simulink model "plant_test"  (R2023b)
settings: Solver=VariableStepAuto  StartTime=0.0  StopTime=t_end  RelTol=1e-3
values from neighbouring files (symbols this model uses):
  param = plant_param()    [plot_bode.m]    (also in plot_impulse.m; plot_initial.m)
  Ts = (2*pi)/(100*w)    [plot_bode.m]    (also in plot_impulse.m = 0.001; plot_initial.m = 0.001)
  w = w_vec(i)    [plot_bode.m]
  x0 = [0;0;10e3;10e3]    [plot_initial.m]
undefined symbols (not defined in the file or in its folder): ue, xe
libraries: fl_lib x32, nesl_utility x14, simulink x4
(part 1 of 3)
settings Model: Creator=MPC5  LastModifiedBy=MPC5

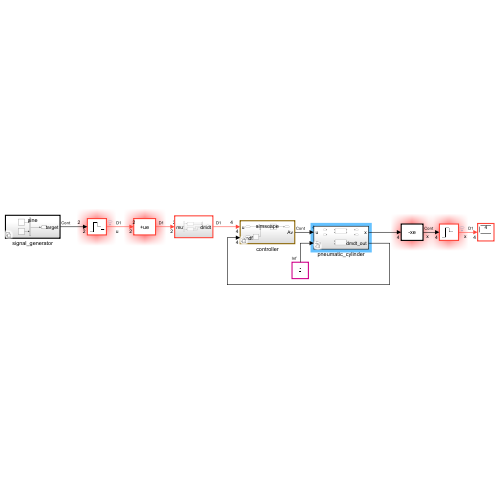
[thumbnail: Simulink's stored preview of the top-level diagram]
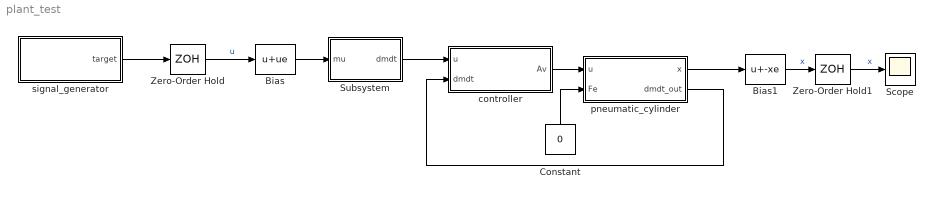
== system plant_test ==
  Bias : Bias  Bias=ue  SaturateOnIntegerOverflow=off
  Bias1 : Bias  Bias=-xe  SaturateOnIntegerOverflow=off
  Constant : Constant  Value=0
  Scope : Scope
  Subsystem : Subsystem
  Zero-Order Hold : ZeroOrderHold  SampleTime=Ts
  Zero-Order Hold1 : ZeroOrderHold  SampleTime=Ts
  controller : Subsystem  Variant=on
  pneumatic_cylinder : Subsystem  Variant=on
  signal_generator : Subsystem  Variant=on
  wires:
  Zero-Order Hold/1 -> Bias/1  "u"
  Bias/1 -> Subsystem/1(mu)
  Subsystem/1(dmdt) -> controller/1(u)
  pneumatic_cylinder/2(dmdt_out) -> controller/2(dmdt)
  controller/1(Av) -> pneumatic_cylinder/1(u)
  Constant/1 -> pneumatic_cylinder/2(Fe)
  pneumatic_cylinder/1(x) -> Bias1/1
  Zero-Order Hold1/1 -> Scope/1  "x"
  signal_generator/1(target) -> Zero-Order Hold/1
  Bias1/1 -> Zero-Order Hold1/1  "x"

== system plant_test/Subsystem ==
  mu : Inport
  Demux : Demux  Outputs=2
  Mux : Mux
  muc_to_dmcdt : Subsystem
  muh_to_dmhdt : Subsystem
  dmdt : Outport
  wires:
  Demux/1 -> muc_to_dmcdt/1(mu)
  muc_to_dmcdt/1(dmdt_in) -> Mux/1
  muc_to_dmcdt/2(dmdt_out) -> Mux/2
  Demux/2 -> muh_to_dmhdt/1(mu)
  muh_to_dmhdt/1(dmdt_in) -> Mux/3
  muh_to_dmhdt/2(dmdt_out) -> Mux/4
  mu/1 -> Demux/1
  Mux/1 -> dmdt/1

== system plant_test/controller ==
  u : Inport
  dmdt : Inport  Port=2
  ode : Subsystem  VariantControl="plant_model_type==\"ode\""
  simscape : Subsystem  VariantControl="plant_model_type==\"simscape\""
  Av : Outport

== system plant_test/pneumatic_cylinder ==
  u : Inport
  Fe : Inport  Port=2
  ode : Subsystem  VariantControl="plant_model_type==\"ode\""
  simscape : Subsystem  VariantControl="plant_model_type==\"simscape\""
  x : Outport
  dmdt_out : Outport  Port=2

== system plant_test/signal_generator ==
  impulse : Subsystem  VariantControl="input_signal_type==\"impulse\""
  sine : Subsystem  VariantControl="input_signal_type==\"sine\""
  zero : Subsystem  VariantControl="input_signal_type==\"zero\""
  target : Outport

== system plant_test/Subsystem/muc_to_dmcdt ==
  note: Pa <= P <= Ps
  mu : Inport
  Constant : Constant  Value=0
  Gain : Gain  Gain=-1
  Gain3 : Gain  Gain=1/param.alpha_in
  Gain4 : Gain  Gain=1/param.alpha_out
  Max : MinMax  Function=max  Inputs=2
  Min : MinMax  Function=max  Inputs=2
  dmdt_in : Outport
  dmdt_out : Outport  Port=2
  wires:
  Gain3/1 -> Max/1
  Constant/1 -> Max/2, Min/1
  Gain/1 -> Gain4/1
  mu/1 -> Gain3/1, Gain/1  "mu"
  Gain4/1 -> Min/2
  Min/1 -> dmdt_out/1  "dmdt_out"
  Max/1 -> dmdt_in/1  "dmdt_in"

== system plant_test/Subsystem/muh_to_dmhdt ==
  note: Pa <= P <= Ps
  mu : Inport
  Constant : Constant  Value=0
  Gain : Gain  Gain=-1
  Gain3 : Gain  Gain=1/param.alpha_in
  Gain4 : Gain  Gain=1/param.alpha_out
  Max : MinMax  Function=max  Inputs=2
  Min : MinMax  Function=max  Inputs=2
  dmdt_in : Outport
  dmdt_out : Outport  Port=2
  wires:
  Gain3/1 -> Max/1
  Constant/1 -> Max/2, Min/1
  Gain/1 -> Gain4/1
  mu/1 -> Gain3/1, Gain/1  "mu"
  Gain4/1 -> Min/2
  Min/1 -> dmdt_out/1  "dmdt_out"
  Max/1 -> dmdt_in/1  "dmdt_in"

== system plant_test/controller/ode ==
  u : Inport  PortDimensions=param.udim
  dmdt : Inport  Port=2  PortDimensions=param.udim
  Terminator : Terminator
  Av : Outport  PortDimensions=param.xdim
  wires:
  u/1 -> Av/1
  dmdt/1 -> Terminator/1

== system plant_test/controller/simscape ==
  u : Inport
  dmdt : Inport  Port=2
  Sum : Sum  Inputs=|+-
  flow rate controller : Subsystem
  Av : Outport
  wires:
  Sum/1 -> flow rate controller/1(e)
  u/1 -> Sum/1
  flow rate controller/1(Av) -> Av/1
  dmdt/1 -> Sum/2

== system plant_test/pneumatic_cylinder/ode ==
  u : Inport
  Fe : Inport  Port=2
  Integrator : Integrator  InitialCondition=x0  LimitOutput=on  UpperSaturationLimit=[param.L/2;inf;inf;inf]  LowerSaturationLimit=[-param.L/2;-inf;-inf;-inf]
  MATLAB Function : MATLAB Function  TreatAsAtomicUnit=on
  Terminator : Terminator
  saturation : Subsystem
  x : Outport
  dmdt_out : Outport  Port=2
  wires:
  saturation/1(u) -> dmdt_out/1, MATLAB Function/2(u)
  Integrator/1 -> x/1, MATLAB Function/1(x), saturation/1(x)
  u/1 -> saturation/2(ud)
  MATLAB Function/1(dxdt) -> Integrator/1
  Fe/1 -> Terminator/1
